simulink model "Propagator"  (R2019a)
settings: Solver=VariableStepAuto  StartTime=0.0  StopTime=10.0  RelTol=1e-3
values from neighbouring files (symbols this model uses):
  JD = jday(Yr,Month,Day,Hr,Min,Sec)    [sgp4_test.m]
(part 1 of 2)
settings Model: Creator=mario  LastModifiedBy=mario

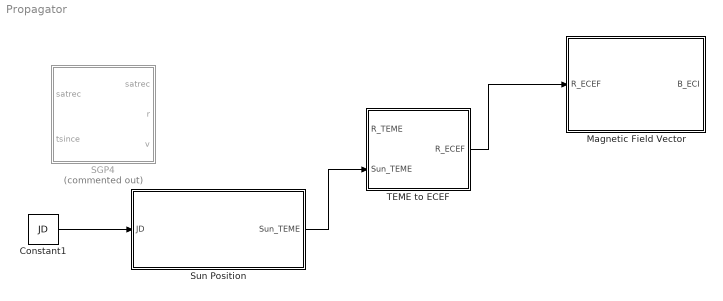
== system Propagator ==
  Constant1 : Constant  Value=JD
  Magnetic Field Vector : Subsystem
  SGP4 : MATLAB Function  Commented=on  TreatAsAtomicUnit=on
  Sun Position : Subsystem
  TEME to ECEF : Subsystem
  wires:
  TEME to ECEF/1(R_ECEF) -> Magnetic Field Vector/1(R_ECEF)
  Constant1/1 -> Sun Position/1(JD)
  Sun Position/1(Sun_TEME) -> TEME to ECEF/2(Sun_TEME)

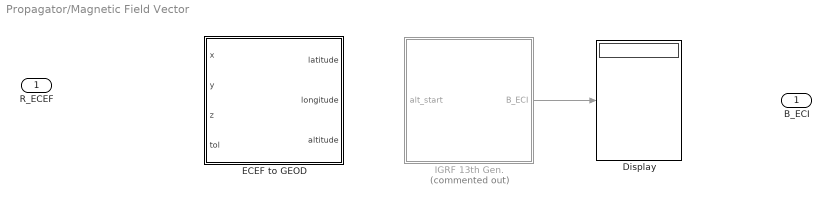
== system Propagator/Magnetic Field Vector ==
  R_ECEF : Inport
  Display : Display
  ECEF to GEOD : MATLAB Function  TreatAsAtomicUnit=on
  IGRF 13th Gen. : MATLAB Function  Commented=on  TreatAsAtomicUnit=on
  B_ECI : Outport
  wires:
  IGRF 13th Gen./1(B_ECI) -> Display/1

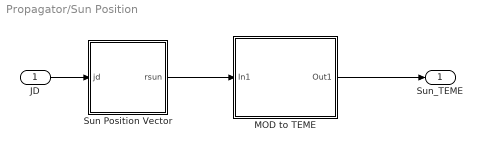
== system Propagator/Sun Position ==
  JD : Inport
  MOD to TEME : Subsystem
  Sun Position Vector : MATLAB Function  TreatAsAtomicUnit=on
  Sun_TEME : Outport
  wires:
  Sun Position Vector/1(rsun) -> MOD to TEME/1(In1)
  JD/1 -> Sun Position Vector/1(jd)
  MOD to TEME/1(Out1) -> Sun_TEME/1

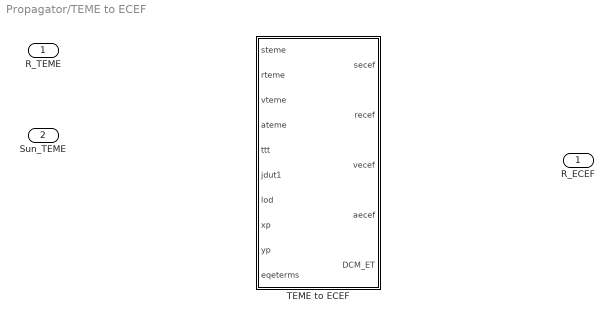
== system Propagator/TEME to ECEF ==
  R_TEME : Inport
  Sun_TEME : Inport  Port=2
  TEME to ECEF : MATLAB Function  TreatAsAtomicUnit=on
  R_ECEF : Outport

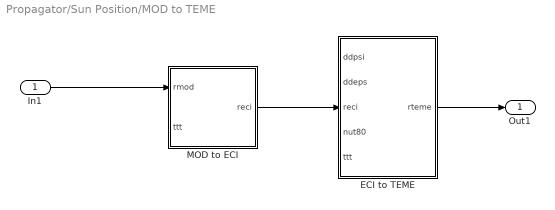
== system Propagator/Sun Position/MOD to TEME ==
  In1 : Inport
  ECI to TEME : MATLAB Function  TreatAsAtomicUnit=on
  MOD to ECI : MATLAB Function  TreatAsAtomicUnit=on
  Out1 : Outport
  wires:
  MOD to ECI/1(reci) -> ECI to TEME/3(reci)
  ECI to TEME/1(rteme) -> Out1/1
  In1/1 -> MOD to ECI/1(rmod)

== matlab function Propagator/SGP4 ==
  data: satrec input; satrec output; tsince input; r output; v output
% -----------------------------------------------------------------------------
%
%                              procedure sgp4
%
%  this procedure is the sgp4 prediction model from space command. this is an
%    updated and combined version of sgp4 and sdp4, which were originally
%    published separately in spacetrack report #3. this version follows the
%    methodology from the aiaa paper (2006) describing the history and
%    development of the code.
%
% Author: 
%   Jeff Beck 
%   beckja@alumni.lehigh.edu
%    current :
%               7 may 08  david vallado
%                           update small eccentricity check
%    changes :
%              16 nov 07  david vallado
%                           misc fixes for better compliance
%   1.0 (aug 7, 2006) - update for paper dav
% original comments from Vallado C++ version:
%   author        : david vallado                  719-573-2600   28 jun 2005
%
%   inputs        :
%     satrec    - initialised structure from sgp4init() call.
%     tsince    - time since epoch (minutes)
%
%   outputs       :
%     r           - position vector                     km
%     v           - velocity                            km/sec
%     return code - non-zero on error.
%                    1 - mean elements, ecc >= 1.0 or ecc < -0.001 or a < 0.95 er
%                    2 - mean motion less than 0.0
%                    3 - pert elements, ecc < 0.0  or  ecc > 1.0
%                    4 - semi-latus rectum < 0.0
%                    5 - epoch elements are sub-orbital
%                    6 - satellite has decayed
%
%   locals        :
%     am          -
%     axnl, aynl        -
%     betal       -
%     COSIM   , SINIM   , COSOMM  , SINOMM  , Cnod    , Snod    , Cos2u   ,
%     Sin2u   , Coseo1  , Sineo1  , Cosi    , Sini    , Cosip   , Sinip   ,
%     Cosisq  , Cossu   , Sinsu   , Cosu    , Sinu
%     Delm        -
%     Delomg      -
%     Dndt        -
%     Eccm        -
%     EMSQ        -
%     Ecose       -
%     El2         -
%     Eo1         -
%     Eccp        -
%     Esine       -
%     Argpm       -
%     Argpp       -
%     Omgadf      -
%     Pl          -
%     R           -
%     RTEMSQ      -
%     Rdotl       -
%     Rl          -
%     Rvdot       -
%     Rvdotl      -
%     Su          -
%     T2  , T3   , T4    , Tc
%     Tem5, Temp , Temp1 , Temp2  , Tempa  , Tempe  , Templ
%     U   , Ux   , Uy    , Uz     , Vx     , Vy     , Vz
%     inclm       - inclination
%     mm          - mean anomaly
%     nm          - mean motion
%     nodem      - longi of ascending node
%     xinc        -
%     xincp       -
%     xl          -
%     xlm         -
%     mp          -
%     xmdf        -
%     xmx         -
%     xmy         -
%     nodedf     -
%     xnode       -
%     nodep      -
%     np          -
%
%   coupling      :
%     getgravconst
%     dpper
%     dspace
%
%   references    :
%     hoots, roehrich, norad spacetrack report #3 1980
%     hoots, norad spacetrack report #6 1986
%     hoots, schumacher and glover 2004
%     vallado, crawford, hujsak, kelso  2006
%  ----------------------------------------------------------------------------*/

function [satrec, r, v] = sgp4(satrec, tsince)

   % /* ------------------ set mathematical constants --------------- */
   twopi = 2.0 * pi;
   x2o3  = 2.0 / 3.0;
   % sgp4fix divisor for divide by zero check on inclination
   % the old check used 1.0 + cos(pi-1.0e-9), but then compared it to
   % 1.5 e-12, so the threshold was changed to 1.5e-12 for consistancy
   temp4    =   1.5e-12;

   %  // sgp4fix identify constants and allow alternate values
   % no longer needed, pass in through satrec
   %global tumin mu radiusearthkm xke j2 j3 j4 j3oj2  
   vkmpersec     = satrec.radiusearthkm * satrec.xke/60.0;
   
   % /* --------------------- clear sgp4 error flag ----------------- */
   satrec.t     = tsince;
   satrec.error = 0;
   mrt = 0.0;

   % /* ------- update for secular gravity and atmospheric drag ----- */
   xmdf    = satrec.mo + satrec.mdot * satrec.t;
   argpdf  = satrec.argpo + satrec.argpdot * satrec.t;
   nodedf  = satrec.nodeo + satrec.nodedot * satrec.t;
   argpm   = argpdf;
   mm      = xmdf;
   t2      = satrec.t * satrec.t;
   nodem   = nodedf + satrec.nodecf * t2;
   tempa   = 1.0 - satrec.cc1 * satrec.t;
   tempe   = satrec.bstar * satrec.cc4 * satrec.t;
   templ   = satrec.t2cof * t2;

   if (satrec.isimp ~= 1)
       delomg = satrec.omgcof * satrec.t;
       delm   = satrec.xmcof *...
           ((1.0 + satrec.eta * cos(xmdf))^3 -...
           satrec.delmo);
       temp   = delomg + delm;
       mm     = xmdf + temp;
       argpm  = argpdf - temp;
       t3     = t2 * satrec.t;
       t4     = t3 * satrec.t;
       tempa  = tempa - satrec.d2 * t2 - satrec.d3 * t3 -...
           satrec.d4 * t4;
       tempe  = tempe + satrec.bstar * satrec.cc5 * (sin(mm) -...
           satrec.sinmao);
       templ  = templ + satrec.t3cof * t3 + t4 * (satrec.t4cof +...
           satrec.t * satrec.t5cof);
   end

   nm    = satrec.no;
   em    = satrec.ecco;
   inclm = satrec.inclo;
   if (satrec.method == 'd')
       tc = satrec.t;
       [satrec.atime,em,argpm,inclm,satrec.xli,mm,...
           satrec.xni,nodem,dndt,nm] = dspace(...
           satrec.d2201,satrec.d2211,satrec.d3210,...
           satrec.d3222,satrec.d4410,satrec.d4422,...
           satrec.d5220,satrec.d5232,satrec.d5421,...
           satrec.d5433,satrec.dedt,satrec.del1,...
           satrec.del2,satrec.del3,satrec.didt,...
           satrec.dmdt,satrec.dnodt,satrec.domdt,...
           satrec.irez,satrec.argpo,satrec.argpdot,satrec.t,...
           tc,satrec.gsto,satrec.xfact,satrec.xlamo,satrec.no,...
           satrec.atime,em,argpm,inclm,satrec.xli,mm,...
           satrec.xni,nodem,nm);
   end % // if method = d

   if (nm <= 0.0)
%       fprintf(1,'# error nm %f\n', nm);
       satrec.error = 2;
   end
   am = (satrec.xke / nm)^x2o3 * tempa * tempa;
   nm = satrec.xke / am^1.5;
   em = em - tempe;

   % // fix tolerance for error recognition
   if ((em >= 1.0) || (em < -0.001) || (am < 0.95))
%       fprintf(1,'# error em %f\n', em);
       satrec.error = 1;
   end
%   sgp4fix change test condition for eccentricity
   if (em < 1.0e-6)
       em  = 1.0e-6;
   end
   mm     = mm + satrec.no * templ;
   xlm    = mm + argpm + nodem;
   emsq   = em * em;
   temp   = 1.0 - emsq;
   nodem  = rem(nodem, twopi);
   argpm  = rem(argpm, twopi);
   xlm    = rem(xlm, twopi);
   mm     = rem(xlm - argpm - nodem, twopi);

   % /* ----------------- compute extra mean quantities ------------- */
   sinim = sin(inclm);
   cosim = cos(inclm);

   % /* -------------------- add lunar-solar periodics -------------- */
   ep     = em;
   xincp  = inclm;
   argpp  = argpm;
   nodep  = nodem;
   mp     = mm;
   sinip  = sinim;
   cosip  = cosim;
   if (satrec.method == 'd')
       [ep,xincp,nodep,argpp,mp] = dpper(...
           satrec.e3,satrec.ee2,satrec.peo,...
           satrec.pgho,satrec.pho,satrec.pinco,...
           satrec.plo,satrec.se2,satrec.se3,...
           satrec.sgh2,satrec.sgh3,satrec.sgh4,...
           satrec.sh2,satrec.sh3,satrec.si2,...
           satrec.si3,satrec.sl2,satrec.sl3,...
           satrec.sl4,satrec.t,satrec.xgh2,...
           satrec.xgh3,satrec.xgh4,satrec.xh2,...
           satrec.xh3,satrec.xi2,satrec.xi3,...
           satrec.xl2,satrec.xl3,satrec.xl4,...
           satrec.zmol,satrec.zmos,satrec.inclo,...
           satrec.init,ep,xincp,nodep,argpp,mp, satrec.operationmode);
       if (xincp < 0.0)
           xincp  = -xincp;
           nodep = nodep + pi;
           argpp  = argpp - pi;
       end
       if ((ep < 0.0 ) || ( ep > 1.0))
%           fprintf(1,'# error ep %f\n', ep);
           satrec.error = 3;
       end
   end % // if method = d

   % /* -------------------- long period periodics ------------------ */
   if (satrec.method == 'd')
       sinip =  sin(xincp);
       cosip =  cos(xincp);
       satrec.aycof = -0.5 * satrec.j3oj2 * sinip;
       % // sgp4fix for divide by zero with xinco = 180 deg
       if (abs(cosip+1.0) > 1.5e-12)
           satrec.xlcof = -0.25 * satrec.j3oj2 * sinip * (3.0 + 5.0 * cosip) /...
               (1.0+cosip);
         else
           satrec.xlcof = -0.25 * satrec.j3oj2 * sinip * (3.0 + 5.0 * cosip) /...
               temp4;
       end;
   end
   axnl = ep * cos(argpp);
   temp = 1.0 / (am * (1.0 - ep * ep));
   aynl = ep* sin(argpp) + temp * satrec.aycof;
   xl   = mp + argpp + nodep + temp * satrec.xlcof * axnl;

   % /* --------------------- solve kepler's equation --------------- */
   u    = rem(xl - nodep, twopi);
   eo1  = u;
   tem5 = 9999.9;
   ktr = 1;
   % //   sgp4fix for kepler iteration
   % //   the following iteration needs better limits on corrections
   while (( abs(tem5) >= 1.0e-12) && (ktr <= 10) )
       sineo1 = sin(eo1);
       coseo1 = cos(eo1);
       tem5   = 1.0 - coseo1 * axnl - sineo1 * aynl;
       tem5   = (u - aynl * coseo1 + axnl * sineo1 - eo1) / tem5;
       if(abs(tem5) >= 0.95)
           if tem5 > 0.0
               tem5 = 0.95;
           else
               tem5 = -0.95;
           end
       end
       eo1    = eo1 + tem5;
       ktr = ktr + 1;
   end

   % /* ------------- short period preliminary quantities ----------- */
   ecose = axnl*coseo1 + aynl*sineo1;
   esine = axnl*sineo1 - aynl*coseo1;
   el2   = axnl*axnl + aynl*aynl;
   pl    = am*(1.0-el2);
   if (pl < 0.0)
%       fprintf(1,'# error pl %f\n', pl);
       satrec.error = 4;
       r = [0;0;0];
       v = [0;0;0];
   else
       rl     = am * (1.0 - ecose);
       rdotl  = sqrt(am) * esine/rl;
       rvdotl = sqrt(pl) / rl;
       betal  = sqrt(1.0 - el2);
       temp   = esine / (1.0 + betal);
       sinu   = am / rl * (sineo1 - aynl - axnl * temp);
       cosu   = am / rl * (coseo1 - axnl + aynl * temp);
       su     = atan2(sinu, cosu);
       sin2u  = (cosu + cosu) * sinu;
       cos2u  = 1.0 - 2.0 * sinu * sinu;
       temp   = 1.0 / pl;
       temp1  = 0.5 * satrec.j2 * temp;
       temp2  = temp1 * temp;

       % /* -------------- update for short period periodics ------------ */
       if (satrec.method == 'd')
           cosisq                 = cosip * cosip;
           satrec.con41  = 3.0*cosisq - 1.0;
           satrec.x1mth2 = 1.0 - cosisq;
           satrec.x7thm1 = 7.0*cosisq - 1.0;
       end
       mrt   = rl * (1.0 - 1.5 * temp2 * betal * satrec.con41) +...
           0.5 * temp1 * satrec.x1mth2 * cos2u;
       su    = su - 0.25 * temp2 * satrec.x7thm1 * sin2u;
       xnode = nodep + 1.5 * temp2 * cosip * sin2u;
       xinc  = xincp + 1.5 * temp2 * cosip * sinip * cos2u;
       mvt   = rdotl - nm * temp1 * satrec.x1mth2 * sin2u / satrec.xke;
       rvdot = rvdotl + nm * temp1 * (satrec.x1mth2 * cos2u +...
           1.5 * satrec.con41) / satrec.xke;

       % /* --------------------- orientation vectors ------------------- */
       sinsu =  sin(su);
       cossu =  cos(su);
       snod  =  sin(xnode);
       cnod  =  cos(xnode);
       sini  =  sin(xinc);
       cosi  =  cos(xinc);
       xmx   = -snod * cosi;
       xmy   =  cnod * cosi;
       ux    =  xmx * sinsu + cnod * cossu;
       uy    =  xmy * sinsu + snod * cossu;
       uz    =  sini * sinsu;
       vx    =  xmx * cossu - cnod * sinsu;
       vy    =  xmy * cossu - snod * sinsu;
       vz    =  sini * cossu;

       % /* --------- position and velocity (in km and km/sec) ---------- */
       r(1) = (mrt * ux)* satrec.radiusearthkm;
       r(2) = (mrt * uy)* satrec.radiusearthkm;
       r(3) = (mrt * uz)* satrec.radiusearthkm;
       v(1) = (mvt * ux + rvdot * vx) * vkmpersec;
       v(2) = (mvt * uy + rvdot * vy) * vkmpersec;
       v(3) = (mvt * uz + rvdot * vz) * vkmpersec;
   end % // if pl > 0

       % // sgp4fix for decaying satellites
        if (mrt < 1.0)
   %         printf("# decay condition %11.6f \n",mrt);
            satrec.error = 6;
        end

   global idebug dbgfile
   if idebug
       debug7;
   end

   return;

== matlab function Propagator/Magnetic Field Vector/IGRF 13th Gen. ==
  data: alt_start input; B_ECI output
function B_ECI = fcn(alt_start)
time = datenum([2007 04 2 11 7 18]);
lat = 30; % Geodetic latitudes in degrees.
lon = 330; % Geodetic longitudes in degrees.
alt_start = 0; % Altitude in km.


B_ECI = igrf(time,lat,lon,100 );

== matlab function Propagator/Sun Position/Sun Position Vector ==
  data: jd input; rsun output
% ------------------------------------------------------------------------------
%
%                           function sun
%
%  this function calculates the geocentric equatorial position vector
%    the sun given the julian date.  this is the low precision formula and
%    is valid for years from 1950 to 2050.  accuaracy of apparent coordinates
%    is 0.01  degrees.  notice many of the calculations are performed in
%    degrees, and are not changed until later.  this is due to the fact that
%    the almanac uses degrees exclusively in their formulations.
%
%  author        : david vallado                  719-573-2600   27 may 2002
%
%  revisions
%    vallado     - fix mean lon of sun                            7 mat 2004
%
%  inputs          description                    range / units
%    jd          - julian date in UTC             days from 4713 bc
%
%  outputs       :
%    rsun        - ijk position vector of the sun au
%    rtasc       - right ascension                rad
%    decl        - declination                    rad
%
%  locals        :
%    meanlong    - mean longitude
%    meananomaly - mean anomaly
%    eclplong    - ecliptic longitude
%    obliquity   - mean obliquity of the ecliptic
%    tut1        - julian centuries of ut1 from
%                  jan 1, 2000 12h
%    ttdb        - julian centuries of tdb from
%                  jan 1, 2000 12h
%    hr          - hours                          0 .. 24              10
%    min         - minutes                        0 .. 59              15
%    sec         - seconds                        0.0  .. 59.99          30.00
%    temp        - temporary variable
%    deg         - degrees
%
%  coupling      :
%    none.
%
%  references    :
%    vallado       2007, 281, alg 29, ex 5-1
%
% [rsun,rtasc,decl] = sun ( jd );
% ------------------------------------------------------------------------------

function rsun  = sun ( jd )

        twopi      =     2.0*pi;
        deg2rad    =     pi/180.0;
        show = 'n';
        
        % -------------------------  implementation   -----------------
        % -------------------  initialize values   --------------------
        tut1= ( jd - 2451545.0  )/ 36525.0;

        if show == 'y'
            fprintf(1,'tut1 %14.9f \n',tut1);
        end

        meanlong= 280.460  + 36000.77*tut1;
        meanlong= rem( meanlong,360.0  );  %deg

        ttdb= tut1;
        meananomaly= 357.5277233  + 35999.05034 *ttdb;
        meananomaly= rem( meananomaly*deg2rad,twopi );  %rad
        if ( meananomaly < 0.0  )
            meananomaly= twopi + meananomaly;
        end

        eclplong= meanlong + 1.914666471 *sin(meananomaly) ...
                    + 0.019994643 *sin(2.0 *meananomaly); %deg
        eclplong= rem( eclplong,360.0  );  %deg

        obliquity= 23.439291  - 0.0130042 *ttdb;  %deg

        eclplong = eclplong *deg2rad;
        obliquity= obliquity *deg2rad;

        % --------- find magnitude of sun vector, )   components ------
        magr= 1.000140612  - 0.016708617 *cos( meananomaly ) ...
                              - 0.000139589 *cos( 2.0 *meananomaly );    % in au's
        rsun = zeros(3,1);
        rsun(1)= magr*cos( eclplong );
        rsun(2)= magr*cos(obliquity)*sin(eclplong);
        rsun(3)= magr*sin(obliquity)*sin(eclplong);

        if show == 'y'
            fprintf(1,'meanlon %11.6f meanan %11.6f eclplon %11.6f obli %11.6f \n', ...
                    meanlong,meananomaly/deg2rad,eclplong/deg2rad,obliquity/deg2rad);
            fprintf(1,'rs %11.9f %11.9f %11.9f \n',rsun);
            fprintf(1,'magr %14.7f \n',magr);
        end

        rtasc= atan( cos(obliquity)*tan(eclplong) );

        % --- check that rtasc is in the same quadrant as eclplong ----
        if ( eclplong < 0.0  )
            eclplong= eclplong + twopi;    % make sure it's in 0 to 2pi range
        end
        if ( abs( eclplong-rtasc ) > pi*0.5  )
            rtasc= rtasc + 0.5 *pi*round( (eclplong-rtasc)/(0.5 *pi));
        end
        decl = asin( sin(obliquity)*sin(eclplong) );

== matlab function Propagator/Sun Position/MOD to TEME/MOD to ECI ==
  data: rmod input; reci output; ttt input
% ----------------------------------------------------------------------------
%
%                           function mod2eci
%
%  this function transforms a vector from the mean equator mean equinox of
%    date (mod) to the mean equator mean equinox (j2000) frame.
%
%  author        : david vallado                  719-573-2600   25 jun 2002
%
%  revisions
%    vallado     - consolidate with iau 2000                     14 feb 2005
%
%  inputs          description                    range / units
%    rmod        - position vector of date
%                    mean equator, mean equinox   km
%    vmod        - velocity vector of date
%                    mean equator, mean equinox   km/s
%    amod        - acceleration vector of date
%                    mean equator, mean equinox   km/s2
%    ttt         - julian centuries of tt         centuries
%
%  outputs       :
%    reci        - position vector eci            km
%    veci        - velocity vector eci            km/s
%    aeci        - acceleration vector eci        km/s2
%
%  locals        :
%    none.
%
%  coupling      :
%   precess      - rotation for precession        mod - eci
%
%  references    :
%    vallado       2001, 219-220, eq 3-68
%
% [reci,veci,aeci] = mod2eci  ( rmod,vmod,amod,ttt );
% ----------------------------------------------------------------------------

function reci  = mod2eci  ( rmod,ttt )
        
        
        [prec,psia,wa,ea,xa] = precess ( ttt);

        reci = prec*rmod;
        
        
        
        
        % ----------------------------------------------------------------------------
%
%                           function precess
%
%  this function calulates the transformation matrix that accounts for the effects
%    of precession. both the 1980 and 2000 theories are handled. note that the 
%    required parameters differ a little. 
%
%  author        : david vallado                  719-573-2600   25 jun 2002
%
%  revisions
%    vallado     - consolidate with iau 2000                     14 feb 2005
%
%  inputs          description                    range / units
%    ttt         - julian centuries of tt
%    opt         - method option                  '01', '02', '96', '80'
%
%  outputs       :
%    prec        - transformation matrix for mod - j2000 (80 only)
%    psia        - cannonical precession angle    rad    (00 only)
%    wa          - cannonical precession angle    rad    (00 only)
%    ea          - cannonical precession angle    rad    (00 only)
%    xa          - cannonical precession angle    rad    (00 only)
%
%  locals        :
%    ttt2        - ttt squared
%    ttt3        - ttt cubed
%    zeta        - precession angle               rad
%    z           - precession angle               rad
%    theta       - precession angle               rad
%    oblo        - obliquity value at j2000 epoch "%
%
%  coupling      :
%    none        -
%
%  references    :
%    vallado       2004, 214-216, 219-221
%
% [prec,psia,wa,ea,xa] = precess ( ttt, opt );
% ----------------------------------------------------------------------------

function [prec,psia,wa,ea,xa] = precess ( ttt );

       % sethelp;
        
        % " to rad
        convrt = pi / (180.0*3600.0);
        ttt2= ttt * ttt;
        ttt3= ttt2 * ttt;

        % ------------------- fk4 b1950 precession angles --------------------
%         if (opt == '50')
% 
%             % ---- Seidelmann pg 107             
%             % for these calls, ttt will come in with the current jd
% %            t1= 0.0; %(ttt - 2433282.42345905)/365242.198782;  % set start as B1850, 0.0 to simplify
% %            t2= (ttt - 2396758.203)/365242.198782;  % uses B1850
% %            ttt = t2 - t1;
% %            ttt2 = ttt * ttt;
% %            ttt3 = ttt * ttt2;
% %            fprintf(1,'50prec %15.9f  \n',ttt);
%             % exp supp 61 pg 38
% %            psia = 50.3708 + 0.0050 * ttt;
% %            wa = 0.0;
% %            ea = 0.0;
% %            xa = 0.1247 - 0.0188 * ttt;
% %            zeta =  (23035.545 + 139.720*t1 + 0.060 *t1*t1)*ttt + (30.240-0.270*t1)*ttt2 + 17.995*ttt3; % "
% %            theta=  (20051.12 - 85.29*t1 - 0.37 *t1*t1)*ttt + (-42.65-0.37*t1)*ttt2 - 41.80*ttt3;
% %            z    =  (23035.545 + 139.720*t1 + 0.060 *t1*t1)*ttt + (109.480+0.390*t1)*ttt2 + 18.325*ttt3;
% 
%             % ---- Newcomb Exp Supp 61 approach, but see GTDS pg 3-17
%             % Exp Supp 61 says use 1900? but gtds says use 1950. 
%             % for these calls, ttt will come in with the current jd
%             t1= 0.0; %(ttt - 2415020.31352)/36524.2198782;  % set start as B1900, 0.0 to simplify
% %            t2= (ttt - 2415020.31352)/36525;  % uses B1900   
%             t2= (ttt - 2433282.42345905)/36525;  % uses B1950  
% %            ttt = t2 - t1;
% %            ttt2 = ttt * ttt;
% %            ttt3 = ttt * ttt2;
%             % exp supp 61 pg 38
%             psia = 50.3708 + 0.0050 * ttt;
%             wa = 0.0; % not sure which one is which...
%             ea = 84428.26 -   46.845*ttt - 0.00059*ttt2 + 0.00181*ttt3;
%             xa = 0.1247 - 0.0188 * ttt;
%            fprintf(1,'50prec %15.9f  \n',ttt);
%            % seems like Exp supp 61 is ok with 1900 as epoch, and Seidlemann is ok with listed measr,  
% %            zeta =  (2304.25 + 1.396*t1)*ttt + 0.302*ttt2 + 0.018*ttt3; % "
% %            theta=  (2004.682 - 0.853*t1)*ttt -0.426*ttt2 - 0.042*ttt3;
% %            z    =  (2304.25 + 1.396*t1)*ttt + 1.093*ttt2 + 0.018*ttt3;
%             % GTDS pg 3-17 using days from 1950 - avoids long rpecession
%             % constants...
%             zeta =  2304.9969*ttt + 0.302*ttt2 + 0.01808*ttt3; % "
%             theta=  2004.2980*ttt -0.425936*ttt2 - 0.0416*ttt3;
%             z    =  2304.9969*ttt + 1.092999*ttt2 + 0.0192*ttt3;
%             
% 
%             % tp-008 36-45
%             % ttt is tropical centruies from 1950 36524.22 days
%             prec = zeros(3,3);
%             prec(1,1) =  1.0 - 2.9696e-4 * ttt2 - 1.3e-7 * ttt3;
%             prec(1,2) =  2.234941e-2 * ttt + 6.76e-6 * ttt2 - 2.21e-6 * ttt3;
%             prec(1,3) =  9.7169e-3 * ttt - 2.07e-6 * ttt2 - 9.6e-7 * ttt3;
%             prec(2,1) =  -prec(1,2);
%             prec(2,2) =  1.0 - 2.4975e-4 * ttt2 - 1.5e-7 * ttt3;
%             prec(2,3) =  - 1.0858e-4 * ttt2;
%             prec(3,1) =  -prec(1,3);
%             prec(3,2) =  prec(2,3);
%             prec(3,3) =  1.0 - 4.721e-5 * ttt2;
%  
%             
%            % pass these back out for testing
%            psia = zeta;
%            wa = theta;
%            ea = z;
%         % ------------------- iau 76 precession angles --------------------
%         else
%           if (opt == '80')
%     fprintf(1,'80prec %15.9f  \n',ttt);
            psia =             5038.7784*ttt - 1.07259*ttt2 - 0.001147*ttt3; % "
            wa   = 84381.448                 + 0.05127*ttt2 - 0.007726*ttt3;
            ea   = 84381.448 -   46.8150*ttt - 0.00059*ttt2 + 0.001813*ttt3;
            xa   =               10.5526*ttt - 2.38064*ttt2 - 0.001125*ttt3;
            zeta =             2306.2181*ttt + 0.30188*ttt2 + 0.017998*ttt3; % "
            theta=             2004.3109*ttt - 0.42665*ttt2 - 0.041833*ttt3;
            z    =             2306.2181*ttt + 1.09468*ttt2 + 0.018203*ttt3;
          % ------------------ iau 03 precession angles -------------------
%           else
%             oblo =  84381.406; % "
%             psia =  (((( -0.0000000951 * ttt + 0.000132851 ) * ttt - 0.00114045 ) * ttt - 1.0790069 ) * ttt + 5038.481507 ) * ttt; % "
%             wa   =  ((((  0.0000003337 * ttt - 0.000000467 ) * ttt - 0.00772503 ) * ttt + 0.0512623 ) * ttt -    0.025754 ) * ttt + oblo;
%             ea   =  (((( -0.0000000434 * ttt - 0.000000576 ) * ttt + 0.00200340 ) * ttt - 0.0001831 ) * ttt -   46.836769 ) * ttt + oblo;
%             xa   =  (((( - 0.0000000560 * ttt + 0.000170663 ) * ttt - 0.00121197 ) * ttt - 2.3814292 ) * ttt +   10.556403 ) * ttt;
% 
%             zeta =  (((( - 0.0000003173 * ttt - 0.000005971 ) * ttt + 0.01801828 ) * ttt + 0.2988499 ) * ttt + 2306.083227 ) * ttt + 2.650545; % "
%             theta=  (((( - 0.0000001274 * ttt - 0.000007089 ) * ttt - 0.04182264 ) * ttt - 0.4294934 ) * ttt + 2004.191903 ) * ttt;
%             z    =  ((((   0.0000002904 * ttt - 0.000028596 ) * ttt + 0.01826837 ) * ttt + 1.0927348 ) * ttt + 2306.077181 ) * ttt - 2.650545;
%           end;
%         end;
        
        % convert units to rad
        psia = psia  * convrt; % rad
        wa   = wa    * convrt;
        ea   = ea    * convrt;
        xa   = xa    * convrt;
        zeta = zeta  * convrt; 
        theta= theta * convrt;
        z    = z     * convrt;
%iauhelp='y';         
%fprintf(1,'pr %11.7f  %11.7f  %11.7fdeg \n',zeta*180/pi,theta*180/pi,z*180/pi );
%         if (iauhelp == 'y')
%             fprintf(1,'pr %11.7f  %11.7f  %11.7f %11.7fdeg \n',psia*180/pi,wa*180/pi,ea*180/pi,xa*180/pi );
%             fprintf(1,'pr %11.7f  %11.7f  %11.7fdeg \n',zeta*180/pi,theta*180/pi,z*180/pi );
%         end;
% 
%         if (strcmp(opt,'80')==1) % || (strcmp(opt,'50') == 1)
            coszeta  = cos(zeta);
            sinzeta  = sin(zeta);
            costheta = cos(theta);
            sintheta = sin(theta);
            cosz     = cos(z);
            sinz     = sin(z);

            % ----------------- form matrix  mod to j2000 -----------------
            prec = zeros(3,3);
            prec(1,1) =  coszeta * costheta * cosz - sinzeta * sinz;
            prec(1,2) =  coszeta * costheta * sinz + sinzeta * cosz;
            prec(1,3) =  coszeta * sintheta;
            prec(2,1) = -sinzeta * costheta * cosz - coszeta * sinz;
            prec(2,2) = -sinzeta * costheta * sinz + coszeta * cosz;
            prec(2,3) = -sinzeta * sintheta;
            prec(3,1) = -sintheta * cosz;
            prec(3,2) = -sintheta * sinz;
            prec(3,3) =  costheta;
